simulink model "s0905"  (Simulink 6.0)
settings: Solver=ode3  SolverMode=SingleTasking  StartTime=0.0  StopTime=900  FixedStep=1  MaxStep=1  RelTol=1e-3  AbsTol=1e-6
undefined symbols (not defined in the file or in its folder): rnen, rzae, snen, szae, wdachrad
settings Model: LastModifiedBy=Froriep
settings DataIOCC: LimitDataPoints=off  SaveOutput=off  TimeSaveName=t
settings OptimizationCC: BooleanDataType=off
settings DebuggingCC: SolverPrmCheckMsg=none
settings HardwareCC: TargetUnknown=on
settings STFCustomTargetCC: TargetFcnLib=ansi_tfl_tmw.mat  GenFloatMathFcnCalls=ANSI_C  ModelReferenceCompliant=off  SystemTargetFile=grt.tlc

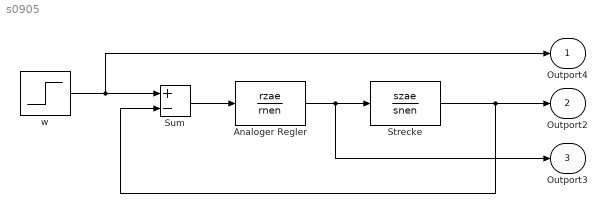
== system s0905 ==
  Analoger Regler : TransferFcn  Numerator=rzae  Denominator=rnen
      mask Display: disp('Gr(s)')
  Strecke : TransferFcn  Numerator=szae  Denominator=snen
      mask Display: disp('Gs(s)')
  Sum : Sum  Inputs=+-  SaturateOnIntegerOverflow=on  InputSameDT=on
  w : Step  Time=.01e-3  After=wdachrad  SampleTime=0
  Outport4 : Outport  InitialOutput=0
  Outport2 : Outport  Port=2  InitialOutput=0
  Outport3 : Outport  Port=3  InitialOutput=0
  wires:
  w/1 -> Outport4/1, Sum/1
  Analoger Regler/1 -> Outport3/1, Strecke/1
  Strecke/1 -> Sum/2, Outport2/1
  Sum/1 -> Analoger Regler/1
